simulink model "solar200W"  (R2020a)
settings: Solver=VariableStepAuto  StartTime=0.0  StopTime=2  RelTol=1e-3
libraries: powerlib x6, re_lib x1
settings Model: Creator=Reaga  LastModifiedBy=Reaga
settings DebuggingCC: UnconnectedInputMsg=none  UnconnectedOutputMsg=none  UnconnectedLineMsg=none
settings ModelReferenceCC: EnableRefExpFcnMdlSchedulingChecks=off
settings RTWCC: Description=Generic Real-Time Target
settings ConfigComp: CovBoundaryAbsTol=1.0e-5

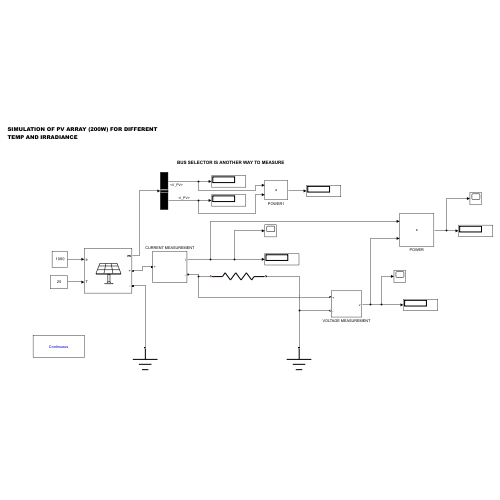
[thumbnail: Simulink's stored preview of the top-level diagram]
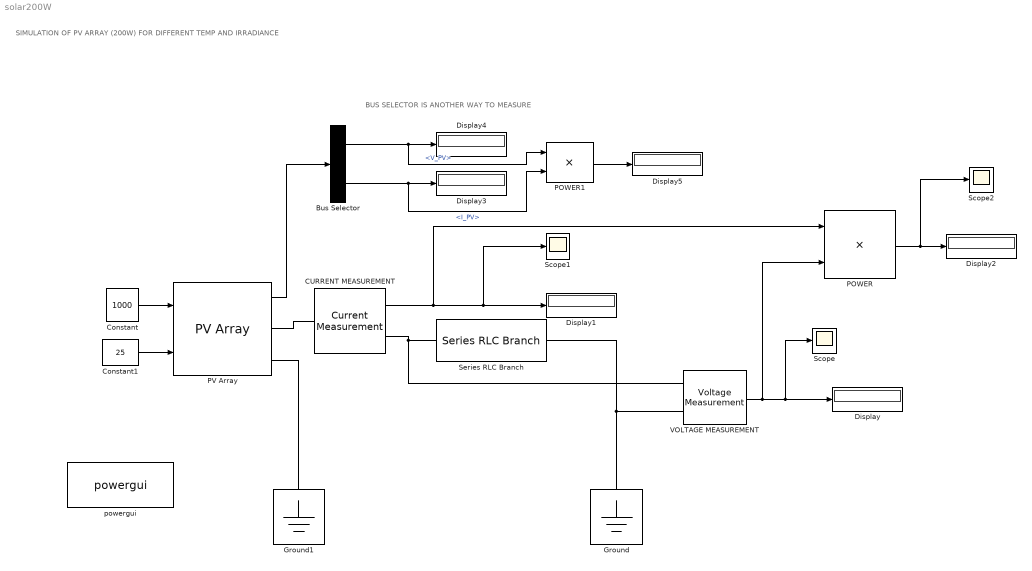
== system solar200W ==
  note: BUS SELECTOR IS ANOTHER WAY TO MEASURE
  note: SIMULATION OF PV ARRAY (200W) FOR DIFFERENT TEMP AND IRRADIANCE
  Bus Selector : BusSelector  OutputSignals=V_PV,I_PV
  CURRENT MEASUREMENT : powerlib/Measurements/Current Measurement  PhasorSimulation=off  OutputType=Complex  PSBequivalent=0
  Constant : Constant  Value=1000
  Constant1 : Constant  Value=25
  Display{,1..5} (6 alike) : Display
  Ground : powerlib/Elements/Ground  LConnTagsString=a
  Ground1 : powerlib/Elements/Ground  LConnTagsString=a
  POWER : Product
  POWER1 : Product
  PV Array : re_lib/Solar/PV Array  Npar=1  Nser=1  PlotType=one module @ 25 deg.C & specified irradiances  S_vec="[ 1000  500  100 ]"  Temp_C_vec="[ 45 25  ]"  ModuleName=User-defined  PlotWhenSelected=off  Pm=200.112  Ncell=54  Voc=32.9  Isc=8.21  Vm=26.4  Im=7.58  beta_Voc_pc=-0.36099  alpha_Isc_pc=0.102  beta_Voc=-0.11877  alpha_Isc=0.0083742  IL=8.2311  I0=3.0465e-10  nI=0.98858  Rsh=126.9934  Rs=0.32653  RobustModel=off  RobustCellTemperature=313.3991  BAL=on  Tc=1e-6  Tfilter=5e-5
  Scope : Scope
  Scope1 : Scope
  Scope2 : Scope
  Series RLC Branch : powerlib/Elements/Series RLC Branch  LConnTagsString=__new0  RConnTagsString=__new0  BranchType=R  Resistance=3.48  Inductance=1e-3  SetiL0=off  InitialCurrent=0  Capacitance=1e-6  Setx0=off  InitialVoltage=0  Measurements=None
  VOLTAGE MEASUREMENT : powerlib/Measurements/Voltage Measurement  PhasorSimulation=off  OutputType=Complex  PSBequivalent=0
  powergui : powerlib/powergui  Priority=1  SimulationMode=Continuous  SampleTime=50e-6  frequency=60  Iterations=50  frequencyindice=0  Pbase=100e6  ErrMax=1e-4  UnitsV=kV  UnitsW=MW  buscounter=0  FunctionMessages=off  echomessages=off  EnableUseOfTLC=off  CurrentSourceSwitches=off  DisableSnubberDevices=off  DisableRonSwitches=off  DisableVfSwitches=off  DisplayEquations=off  AutomaticDiscreteSolvers=off  SolverType=Tustin/Backward Euler (TBE)  Interpol=off  ExternalGateDelay=off  methode=off  Ts=100  x0status=blocks  SPID=on  SwTol=0  HookPort=off  NonlinearTolerance=1e-4  nMaxIteration=100  ContinueOnMaxIteration=off  RestoreLinks=warning  ResistiveCurrentMeasurement=off  Frange=[0:2:500]  Ylog=off  Xlog=on  ShowGrid=off  save=off  variable=ZData  structure=0  ZoomFFT=off  StartTime=0.0  cycles=1  DisplayStyle=1  fundamental=60  FreqAxis=off  MaxFrequency=1000  frequencyindicesteady=1  RmsSteady=1  display=off
  wires:
  Constant/1 -> PV Array/1
  Constant1/1 -> PV Array/2
  VOLTAGE MEASUREMENT/1 -> POWER/2, Scope/1, Display/1
  CURRENT MEASUREMENT/1 -> POWER/1, Scope1/1, Display1/1
  POWER/1 -> Scope2/1, Display2/1
  Bus Selector/1 -> POWER1/1, Display4/1  "<V_PV>"
  Bus Selector/2 -> POWER1/2, Display3/1  "<I_PV>"
  PV Array/1 -> Bus Selector/1
  POWER1/1 -> Display5/1
  connections:
  Series RLC Branch/RConn1 -- VOLTAGE MEASUREMENT/LConn2 -- Ground/LConn1
  Ground1/LConn1 -- PV Array/RConn2
  CURRENT MEASUREMENT/LConn1 -- PV Array/RConn1
  Series RLC Branch/LConn1 -- VOLTAGE MEASUREMENT/LConn1 -- CURRENT MEASUREMENT/RConn1
